simulink model "Two_Sine_Phase_Sim"  (R2024b)
settings: Solver=FixedStepAuto  StartTime=0.0  StopTime=2  FixedStep=0.001  RelTol=1e-3
libraries: dspstat3 x1
settings Model: Creator=leoni  LastModifiedBy=leoni

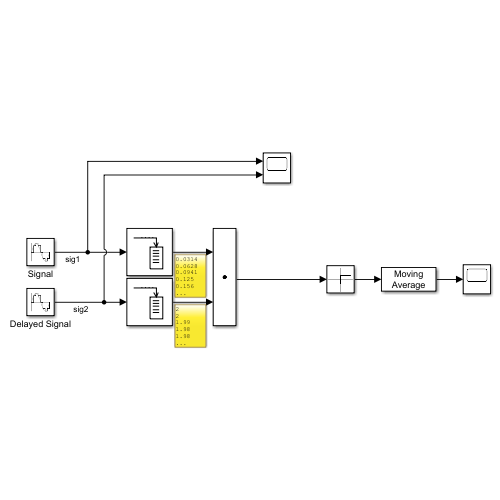
[thumbnail: Simulink's stored preview of the top-level diagram]
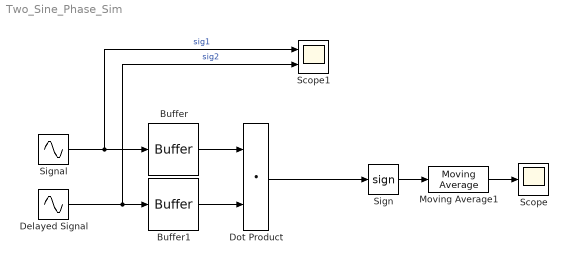
== system Two_Sine_Phase_Sim ==
  Buffer : Buffer  N=200  V=199  OutputFrames=off
  Buffer1 : Buffer  N=200  V=199  OutputFrames=off
  Delayed Signal : Sin  Amplitude=2  Frequency=2*pi*5  Phase=pi/2  SampleTime=0.001  VectorParams1D=off
  Dot Product : DotProduct  OutDataTypeStr=Inherit: Inherit via internal rule
  Moving Average1 : dspstat3/Moving Average  Method=Exponential weighting  ForgettingFactorPort=off  SpecifyWindowLength=on  WindowLength=1000  OverlapLength=10  AllowArbitraryInputLength=off  ForgettingFactor=0.9  SimulateUsing=Interpreted execution
  Scope : Scope
  Scope1 : Scope  NumInputPorts=2
  Sign : Signum
  Signal : Sin  Frequency=2*pi*5  SampleTime=0.001
  wires:
  Signal/1 -> Scope1/1, Buffer/1  "sig1"
  Delayed Signal/1 -> Scope1/2, Buffer1/1  "sig2"
  Buffer/1 -> Dot Product/1
  Buffer1/1 -> Dot Product/2
  Dot Product/1 -> Sign/1
  Sign/1 -> Moving Average1/1
  Moving Average1/1 -> Scope/1
